simulink model "NDO_STO_old"  (R2017b)
settings: Solver=FixedStepAuto  StartTime=0.0  StopTime=100  FixedStep=0.001  RelTol=1e-3
undefined symbols (not defined in the file): B, k1, k10, k11, k12, k2, k3, k4, k5, k6, k7, k8, k9, MI, x5r, x7r
libraries: powerlib_extras x21, commchan3 x15, simulink x3, checkpacklib x2
(part 3 of 3)

== matlab function NDO_STO_old/MATLAB Function ==
  data: x output; dx output; ddx output; t input; y output; dy output; ddy output; z output; dz output; ddz output; yaw output
function [x,dx,ddx,y,dy,ddy,z,dz,ddz,yaw] = desired_trajectory(t)

yaw=0;
if (t>=0 && t<10)
    x=0;
    y=0;
    z=0;
   dx=0;
ddx=0;
dy=0;
ddy=0;
dz=0;
ddz=0;

else
    x=0.5*sin(2.0*pi/10.0*t);
    dx=0.5*2.0*pi/10.0*cos(2.0*pi/10.0*t);
    ddx=-0.5*2.0*pi/10.0*2.0*pi/10.0*sin(2.0*pi/10.0*t);
    
    y=0.5*cos(2.0*pi/10.0*t);
    dy=-0.5*2.0*pi/10.0*sin(2.0*pi/10.0*t);
    ddy=-0.5*2.0*pi/10.0*2.0*pi/10.0*cos(2.0*pi/10.0*t);
    z=1;
    dz=0;
    ddz=0;
    
end

== matlab function NDO_STO_old/Subsystem2/xyz _desired1 ==
  data: x output; t input; y output; z output; dx output; dy output; dz output; ddx output; ddy output; ddz output; yaw output

function [x,y,z,dx,dy,dz,ddx,ddy,ddz,yaw]=traj_vehic(t)

xf1=0;
yf1=0;
zf1=0;
yaw=0;
dxf1=0;
ddxf1=0;
dyf1=0;
ddyf1=0;
dzf1=0;
ddzf1=0;
if t<=10 
    
    x0=0;
    y0=0;
    z0=0;
     
xf=0.2;
yf=0.2;
zf=0.2;

tf=10;
 
a0y=y0;%yf=20;
a1y=0;
a2y=(3/(tf^2))*(yf-y0);
a3y=-(2/(tf^3))*(yf-y0);

a0x=x0;%yf=20;
a1x=0;
a2x=(3/(tf^2))*(xf-x0);
a3x=-(2/(tf^3))*(xf-x0);

a0z=z0;%yf=20;
a1z=0;
a2z=(3/(tf^2))*(zf-z0);
a3z=-(2/(tf^3))*(zf-z0);

 
xf1=a0x+a2x*t^2+a3x*t^3; 
yf1=a0y+a2y*t^2+a3y*t^3;
zf1=a0z+a2z*t^2+a3z*t^3;
dxf1=2*a2x*t+3*a3x*t^2;%1.3*(pi/2.5)*sin(pi*t/2.5);%
ddxf1=2*a2x+2*3*a3x*t;
dyf1=2*a2y*t+3*a3y*t^2;%0.5*(pi/12.5)*cos(pi*t/12.5);%
ddyf1=2*a2y+2*3*a3y*t;
dzf1=2*a2z*t+3*a3x*t^2;
ddzf1=2*a2z+2*3*a3z*t;
end

if t>10 && t<=20
    
 xf1=0.2;
yf1=0.2;
zf1=0.2;
dxf1=0;%1.3*(pi/2.5)*sin(pi*t/2.5);%
ddxf1=0;
dyf1=0;%0.5*(pi/12.5)*cos(pi*t/12.5);%
ddyf1=0;
dzf1=0;
ddzf1=0;
end


if t>20 && t<=30
    yf1=0.2;
    zf1=0.2;
    x0=0.2;
   
    xf=0.3;
    tf=10;
a0x=x0;%yf=20;
a1x=0;
a2x=(3/(tf^2))*(xf-x0);
a3x=-(2/(tf^3))*(xf-x0);

 
xf1=a0x+a2x*(t-20)^2+a3x*(t-20)^3; 
dxf1=2*a2x*(t-20)+3*a3x*(t-20)^2;%1.3*(pi/2.5)*sin(pi*t/2.5);%
ddxf1=2*a2x+2*3*a3x*(t-20);
dyf1=0;
ddyf1=0;
dzf1=0;
ddzf1=0;
end

if t>30 && t<=40

    xf1=0.3;
    zf1=0.2;
    y0=0.2;
    yf=0.3;
    tf=10;     
     
    a0y=y0;%yf=20;
    a1y=0;
    a2y=(3/(tf^2))*(yf-y0);
    a3y=-(2/(tf^3))*(yf-y0);
 
yf1=a0y+a2y*(t-30)^2+a3y*(t-30)^3;

dxf1=0; %2*a2x*(t-40)+3*a3x*(t-40)^2;%1.3*(pi/2.5)*sin(pi*t/2.5);%
ddxf1=0;
dyf1=2*a2y*(t-30)+3*a3y*(t-30)^2;%0.5*(pi/12.5)*cos(pi*t/12.5 
ddyf1=2*a2y+2*3*a3y*(t-30);
dzf1=0;
ddzf1=0;
end 

if t>40 && t<=50
    xf1=0.3;
    yf1=0.3;
    zf1=0.2;
dxf1=0;%2*a2x*(t-55)+3*a3x*(t-55)^2;%1.3*(pi/2.5)*sin(pi*t/2.5);%
ddxf1=0;
dyf1=0;%2*a2y*(t-55)+3*a3y*(t-55)^2;%0.5*(pi/12.5)*cos(pi*t/12.5
ddyf1=0;
dzf1=0;
ddzf1=0;
end

if t>50 && t<=60
    x0=0.3;
    xf=0.2;
    y0=0.3;
    yf=0.2;
    tf=10;
    zf1=0.2;
a0y=y0;%yf=20;
a1y=0;
a2y=(3/(tf^2))*(yf-y0);
a3y=-(2/(tf^3))*(yf-y0);

a0x=x0;%yf=20;
a1x=0;
a2x=(3/(tf^2))*(xf-x0);
a3x=-(2/(tf^3))*(xf-x0);

xf1=a0x+a2x*(t-50)^2+a3x*(t-50)^3; 
yf1=a0y+a2y*(t-50)^2+a3y*(t-50)^3;

dxf1=2*a2x*(t-50)+3*a3x*(t-50)^2;%1.3*(pi/2.5)*sin(pi*t/2.5);%
ddxf1=2*a2x+2*3*a3x*(t-50);
dyf1=2*a2y*(t-50)+3*a3y*(t-50)^2;%0.5*(pi/12.5)*cos(pi*t/12.5 
ddyf1=2*a2y+2*3*a3y*(t-50);
dzf1=0;
ddzf1=0;
end
    
 if t>60  
     
     xf1=0.2;
     yf1=0.2;
     zf1=0.2;
     dxf1=0;
     ddxf1=0;
     dyf1=0;
     ddyf1=0;
     dzf1=0;
     ddzf1=0;
 end    

     

x=xf1;
y=yf1;
z=zf1;
dx=dxf1;
dy=dyf1;
dz=dzf1;
ddx=ddxf1;
ddy=ddyf1;
ddz=ddzf1;
